simulink model "simulink01"  (Simulink 7.7)
settings: Solver=ode45  StartTime=0.0  StopTime=0.1  RelTol=1e-3
values from neighbouring files (symbols this model uses):
  k1 = -(((Ra)/(La))+((B)/(J)))    (= -28739.5050064)    [parametriza_motor.m]
  k2 = -((((Ra)*(B))+((alpha)^2))/((J)*(La)))    (= -280.112044818)    [parametriza_motor.m]
  k3 = ((alpha)/((J)*(La)))    (= 154.758035811)    [parametriza_motor.m]
settings Model: Creator=Felipe  LastModifiedBy=Felipe

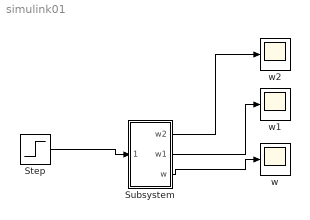
== system simulink01 ==
  Step : Step  Time=0  Before=5  SampleTime=0
  Subsystem : Subsystem
  w : Scope
      settings: SaveName=ScopeData2
  w1 : Scope
  w2 : Scope
  wires:
  Subsystem/3(w) -> w/1
  Step/1 -> Subsystem/1(ei(t))
  Subsystem/1(w2) -> w2/1
  Subsystem/2(w1) -> w1/1

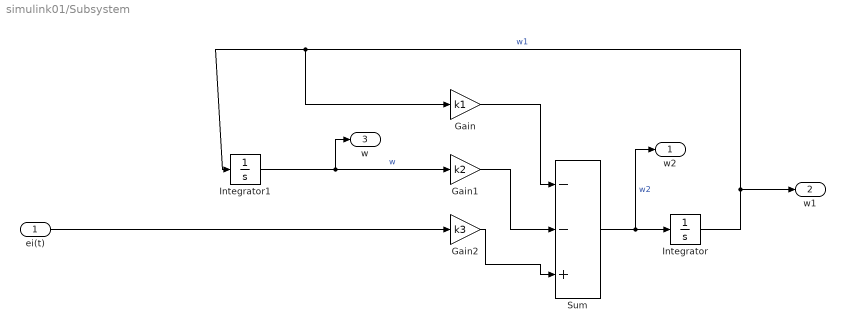
== system simulink01/Subsystem ==
  ei(t) : Inport
  Gain : Gain  Gain=k1
  Gain1 : Gain  Gain=k2
  Gain2 : Gain  Gain=k3
  Integrator : Integrator
  Integrator1 : Integrator
  Sum : Sum  Inputs=--+
  w2 : Outport
  w1 : Outport  Port=2
  w : Outport  Port=3
  wires:
  Gain2/1 -> Sum/3
  Gain/1 -> Sum/1
  Sum/1 -> Integrator/1, w2/1  "w2"
  Integrator/1 -> Gain/1, Integrator1/1, w1/1  "w1"
  Integrator1/1 -> Gain1/1, w/1  "w"
  ei(t)/1 -> Gain2/1
  Gain1/1 -> Sum/2
